simulink model "mongolfiera"  (R2021a)
settings: Solver=VariableStepAuto  StartTime=0.0  StopTime=tsim  RelTol=0.1
values from neighbouring files (symbols this model uses):
  b = 20    [main.m]
  c = 718    [main.m]
  f_w = 0    [main.m]
  g = 9.81    [main.m]
  k = 2.5    [main.m]
  m = 500    [main.m]
  p_a = 1.184    [main.m]
  theta_a = 298    [main.m]
  u_eq = k*(theta - theta_a)    (= 199.411134904)    [main.m]
  V = 2000    [main.m]
  x_eq = [600;0;theta]    [main.m]
settings Model: Creator=Randy  LastModifiedBy=Randy

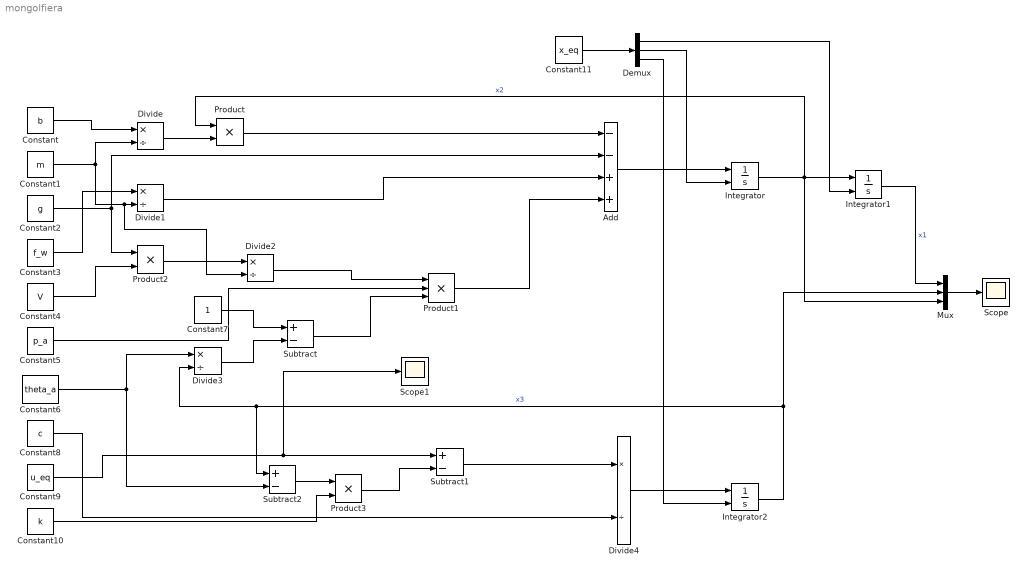
== system mongolfiera ==
  Add : Sum  Inputs=--++
  Constant : Constant  Value=b
  Constant1 : Constant  Value=m
  Constant10 : Constant  Value=k
  Constant11 : Constant  Value=x_eq
  Constant2 : Constant  Value=g
  Constant3 : Constant  Value=f_w
  Constant4 : Constant  Value=V
  Constant5 : Constant  Value=p_a
  Constant6 : Constant  Value=theta_a
  Constant7 : Constant
  Constant8 : Constant  Value=c
  Constant9 : Constant  Value=u_eq
  Demux : Demux  Outputs=3
  Divide{,1..4} (5 alike) : Product  Inputs=*/
  Integrator : Integrator  InitialConditionSource=external
  Integrator1 : Integrator  InitialConditionSource=external  InitialCondition=600
  Integrator2 : Integrator  InitialConditionSource=external  InitialCondition=377
  Mux : Mux  Inputs=3
  Product : Product
  Product1 : Product  Inputs=3
  Product2 : Product
  Product3 : Product
  Scope : Scope
  Scope1 : Scope
  Subtract : Sum  Inputs=+-
  Subtract1 : Sum  Inputs=+-
  Subtract2 : Sum  Inputs=+-
  wires:
  Add/1 -> Integrator/1
  Integrator/1 -> Product/1, Integrator1/1, Mux/3  "x2"
  Constant/1 -> Divide/1
  Constant1/1 -> Divide2/2, Divide1/2, Divide/2
  Divide/1 -> Product/2
  Product/1 -> Add/1
  Constant2/1 -> Product2/1, Add/2
  Constant3/1 -> Divide1/1
  Divide1/1 -> Add/3
  Constant4/1 -> Product2/2
  Product2/1 -> Divide2/1
  Divide2/1 -> Product1/1
  Constant5/1 -> Product1/2
  Divide3/1 -> Subtract/2
  Constant6/1 -> Subtract2/2, Divide3/1
  Integrator2/1 -> Mux/2, Subtract2/1, Divide3/2  "x3"
  Constant7/1 -> Subtract/1
  Subtract/1 -> Product1/3
  Product1/1 -> Add/4
  Divide4/1 -> Integrator2/1
  Constant8/1 -> Divide4/2
  Constant9/1 -> Scope1/1, Subtract1/1
  Product3/1 -> Subtract1/2
  Constant10/1 -> Product3/2
  Subtract2/1 -> Product3/1
  Subtract1/1 -> Divide4/1
  Integrator1/1 -> Mux/1  "x1"
  Mux/1 -> Scope/1
  Constant11/1 -> Demux/1
  Demux/1 -> Integrator1/2
  Demux/2 -> Integrator/2
  Demux/3 -> Integrator2/2
